simulink model "Filter"  (R2014b)
settings: Solver=ode45  StartTime=0.0  StopTime=10.0  RelTol=1e-3
libraries: dsparch4 x2
settings Model: Creator=Karan  LastModifiedBy=Karan

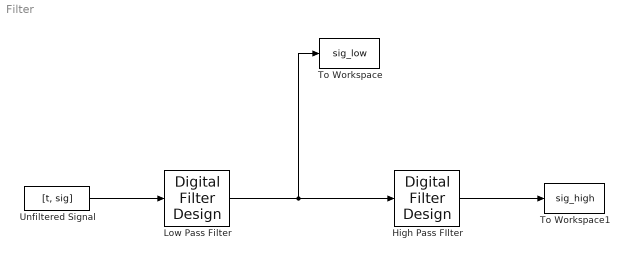
== system Filter ==
  High Pass FIlter : dsparch4/Digital Filter Design  mwdsp_browser_bugfix_var=off
  Low Pass Filter : dsparch4/Digital Filter Design  mwdsp_browser_bugfix_var=off
  To Workspace : ToWorkspace  VariableName=sig_low  SampleTime=1/800
      settings: Save2DSignal=2-D array (concatenate along first dimension)
  To Workspace1 : ToWorkspace  VariableName=sig_high  SampleTime=1/800
      settings: Save2DSignal=2-D array (concatenate along first dimension)
  Unfiltered Signal : FromWorkspace  VariableName=[t, sig]  SampleTime=1/800
  wires:
  Unfiltered Signal/1 -> Low Pass Filter/1
  Low Pass Filter/1 -> High Pass FIlter/1, To Workspace/1
  High Pass FIlter/1 -> To Workspace1/1
